simulink model "abb_pd_g"  (Simulink 10.3)
settings: Solver=ode45  StartTime=0.0  StopTime=inf  RelTol=1e-3
undefined symbols (not defined in the file): abb_eom_solution, abbRobot, control_pd_g, hamiltonian_fun_solution, I_Je_fun_solution
libraries: simulink x7
settings Model: Creator=dario  LastModifiedBy=iansc
settings DataIOCC: LimitDataPoints=on  SignalLoggingSaveFormat=Dataset
settings OptimizationCC: BlockReduction=off  BooleanDataType=off  ExpressionDepthLimit=128
settings DebuggingCC: SaveWithParameterizedLinksMsg=none  SignalResolutionControl=TryResolveAllWithWarning  StateNameClashWarn=none  SFExecutionAtInitializationDiag=warning
settings HardwareCC: TargetUnknown=on
settings GRTTargetCC: CombineOutputUpdateFcns=on  GRTInterface=off

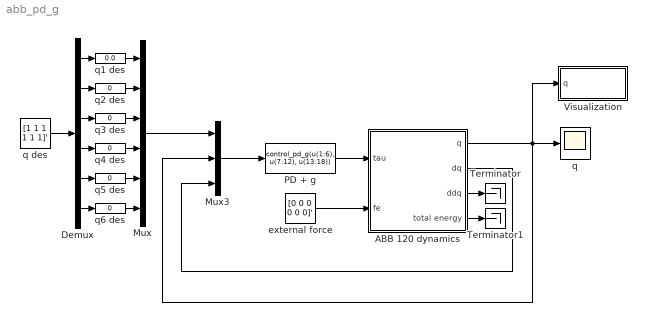
== system abb_pd_g ==
  ABB 120 dynamics : Subsystem  mask{Ts=0.01, F=[0.1 0.1 0.1 0.1 0.1 0.1]', phi0=[0 0 0 0 0 0]', dphi0=[0 0 0 0 0 0]', enable_g=on, enable_f=off}
      mask prompts: Ts "Sample time"; F "Viscous friction (6x1)"; phi0 "Initial joint positions"; dphi0 "Initial joint velocities"; enable_g "Enable gravity"; enable_f "Enable friction"
  Demux : Demux  Outputs=6
  Mux : Mux  Inputs=6
  Mux3 : Mux  Inputs=3
  PD + g : MATLABFcn  MATLABFcn=control_pd_g(u(1:6), u(7:12), u(13:18))  OutputDimensions=[6,1]  Output1D=off
  Terminator : Terminator
  Terminator1 : Terminator
  Visualization : Subsystem
  external force : Constant  Value=[0 0 0 0 0 0]'
  q : Scope
  q des : Constant  Value=[1 1 1 1 1 1]'
  q1 des : simulink/Math Operations/Slider Gain  gain=0.0  low=-2  high=2
  q2 des : simulink/Math Operations/Slider Gain  gain=0  low=-2  high=2
  q3 des : simulink/Math Operations/Slider Gain  gain=0  low=-2  high=2
  q4 des : simulink/Math Operations/Slider Gain  gain=0  low=-2  high=2
  q5 des : simulink/Math Operations/Slider Gain  gain=0  low=-2  high=2
  q6 des : simulink/Math Operations/Slider Gain  gain=0  low=-2  high=2
  wires:
  ABB 120 dynamics/1(q) -> Visualization/1(q), q/1, Mux3/2
  external force/1 -> ABB 120 dynamics/2(fe)
  Mux3/1 -> PD + g/1
  ABB 120 dynamics/2(dq) -> Mux3/3
  PD + g/1 -> ABB 120 dynamics/1(tau)
  ABB 120 dynamics/3(ddq) -> Terminator/1
  ABB 120 dynamics/4(total energy) -> Terminator1/1
  Demux/1 -> q1 des/1
  Demux/2 -> q2 des/1
  Demux/4 -> q4 des/1
  Demux/6 -> q6 des/1
  q6 des/1 -> Mux/6
  q5 des/1 -> Mux/5
  q4 des/1 -> Mux/4
  q3 des/1 -> Mux/3
  q2 des/1 -> Mux/2
  q1 des/1 -> Mux/1
  q des/1 -> Demux/1
  Mux/1 -> Mux3/1
  Demux/3 -> q3 des/1
  Demux/5 -> q5 des/1

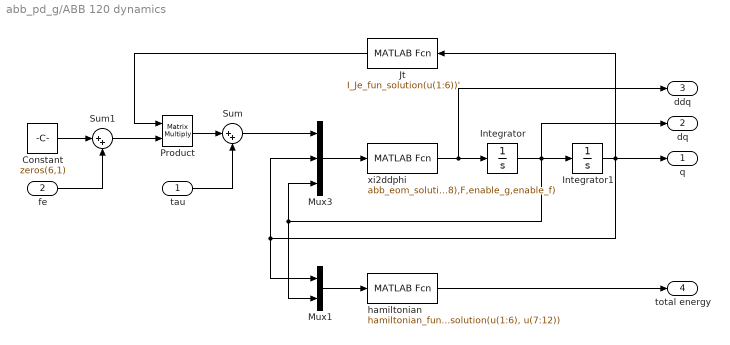
== system abb_pd_g/ABB 120 dynamics ==
  tau : Inport
  fe : Inport  Port=2
  Constant : Constant  Value=zeros(6,1)
  Integrator : Integrator  InitialCondition=dphi0
  Integrator1 : Integrator  InitialCondition=phi0
  Jt : MATLABFcn  MATLABFcn=I_Je_fun_solution(u(1:6))'  OutputDimensions=[6,6]  OutputSignalType=real  Output1D=off
  Mux1 : Mux  Inputs=2
  Mux3 : Mux  Inputs=3
  Product : Product  Multiplication=Matrix(*)
  Sum : Sum  Inputs=|++
  Sum1 : Sum  Inputs=|++
  hamiltonian : MATLABFcn  MATLABFcn=hamiltonian_fun_solution(u(1:6), u(7:12))  OutputDimensions=[1,1]  Output1D=off
  xi2ddphi : MATLABFcn  MATLABFcn=abb_eom_solution(u(1:6), u(7:12), u(13:18),F,enable_g,enable_f)  OutputDimensions=[6,1]  Output1D=off
  q : Outport
  dq : Outport  Port=2
  ddq : Outport  Port=3
  total energy : Outport  Port=4
  wires:
  Integrator/1 -> Mux1/2, Mux3/3, dq/1, Integrator1/1
  tau/1 -> Sum/2
  Integrator1/1 -> Jt/1, Mux1/1, Mux3/2, q/1
  Mux3/1 -> xi2ddphi/1
  xi2ddphi/1 -> ddq/1, Integrator/1
  Mux1/1 -> hamiltonian/1
  hamiltonian/1 -> total energy/1
  Jt/1 -> Product/1
  Product/1 -> Sum/1
  Sum/1 -> Mux3/1
  Constant/1 -> Sum1/1
  fe/1 -> Sum1/2
  Sum1/1 -> Product/2

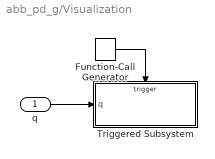
== system abb_pd_g/Visualization ==
  q : Inport
  Function-Call Generator : simulink/Ports & Subsystems/Function-Call Generator  sample_time=0.05  numberOfIterations=1  DisallowWideOutput=off
  Triggered Subsystem : Subsystem  TreatAsAtomicUnit=on
  wires:
  Function-Call Generator/1 -> Triggered Subsystem/Trigger
  q/1 -> Triggered Subsystem/1(q)

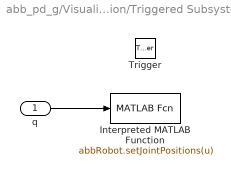
== system abb_pd_g/Visualization/Triggered Subsystem ==
  q : Inport
  Trigger : TriggerPort  TriggerType=function-call  VariantControl=Variant
  Interpreted MATLAB Function : MATLABFcn  MATLABFcn=abbRobot.setJointPositions(u)  OutputDimensions=0
  wires:
  q/1 -> Interpreted MATLAB Function/1
